simulink model "EV3_test"  (Simulink 7.6)
settings: Solver=FixedStepDiscrete  StartTime=0.0  StopTime=Inf  RelTol=1e-3
libraries: rpi_blkst x1
settings Model: Creator=jacques  LastModifiedBy=jacques  SimulationMode=external
settings OptimizationCC: OptimizeModelRefInitCode=on  LifeSpan=1
settings HardwareCC: ProdIntDivRoundTo=Zero  ProdEndianess=LittleEndian  ProdHWDeviceType=Intel->x86/Pentium
settings RTWCC: SystemTargetFile=ert_rpi.tlc  TemplateMakefile=ert_rpi.tmf  PostCodeGenCommand=postGenFunc(buildInfo)  Description=RTW Embedded Coder RPI target  ProcessScript=ert_rpi_make_rtw_hook
settings CodeAppCC: IgnoreCustomStorageClasses=off
settings STFCustomTargetCC: ModelReferenceCompliant=off  CombineOutputUpdateFcns=on  ERTCustomFileBanners=on  SupportNonInlinedSFcns=off  SystemTargetFile=ert_rpi.tlc
settings ERTTargetCC: MultiwordLength=2048  ModelReferenceCompliant=off  ParMdlRefBuildCompliant=off  CompOptLevelCompliant=off  ERTFirstTimeCompliant=off  SupportContinuousTime=on  ModelStepFunctionPrototypeControlCompliant=off  CPPClassGenCompliant=off  ExtMode=on  ExtModeMexArgs='192.168.2.1'  InlinedParameterPlacement=NonHierarchical  ERTCustomFileTemplate=ert_rpi_file_process.tlc  ConvertIfToSwitch=off

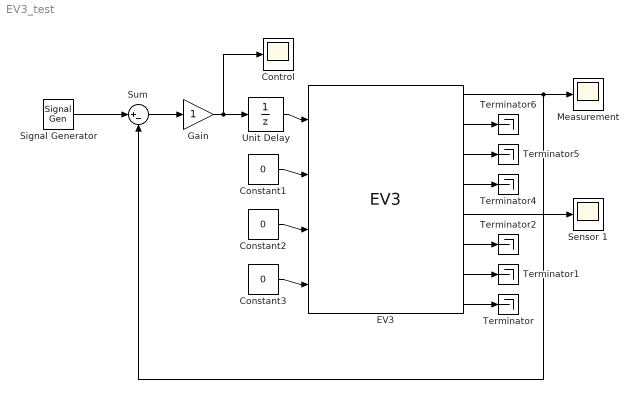
== system EV3_test ==
  Constant1 : Constant  Value=0
  Constant2 : Constant  Value=0
  Constant3 : Constant  Value=0
  Control : Scope
      settings: YMin=-100  YMax=100
  EV3 : rpi_blkst/EV3  SystemSampleTime=-1  rpi_mask_Ts=0.01
  Gain : Gain
  Measurement : Scope
      settings: YMin=-110  YMax=110
  Sensor 1 : Scope
      settings: YMin=85  YMax=165  SaveName=ScopeData2
  Signal Generator : SignalGenerator  WaveForm=square  Amplitude=40  Frequency=0.5
  Sum : Sum  Inputs=|+-
  Terminator{,1..2,4..6} (6 alike) : Terminator
  Unit Delay : UnitDelay  SampleTime=-1
  wires:
  Constant1/1 -> EV3/2
  Constant2/1 -> EV3/3
  Constant3/1 -> EV3/4
  EV3/8 -> Terminator/1
  EV3/7 -> Terminator1/1
  EV3/6 -> Terminator2/1
  EV3/5 -> Sensor 1/1
  EV3/1 -> Measurement/1, Sum/2
  EV3/4 -> Terminator4/1
  EV3/3 -> Terminator5/1
  EV3/2 -> Terminator6/1
  Gain/1 -> Unit Delay/1, Control/1
  Unit Delay/1 -> EV3/1
  Signal Generator/1 -> Sum/1
  Sum/1 -> Gain/1
